simulink model "untitled"  (R2023a)
settings: Solver=VariableStepAuto  StartTime=0.0  StopTime=10.0  RelTol=1e-3
(part 2 of 2)

== system untitled/Subsystem/AdjustingStage/Normalizer/EightBitComparator/FourBitComparator ==
  In1 : Inport
  In2 : Inport  Port=2
  In3 : Inport  Port=3
  In5 : Inport  Port=4
  In4 : Inport  Port=5
  FourBitComparator : Subsystem
  Out1 : Outport
  Out2 : Outport  Port=2
  Out3 : Outport  Port=3

== system untitled/Subsystem/AdjustingStage/Normalizer/EightBitComparator/FourBitComparator1 ==
  In1 : Inport
  In2 : Inport  Port=2
  In3 : Inport  Port=3
  In5 : Inport  Port=4
  In4 : Inport  Port=5
  Out1 : Outport
  Out2 : Outport  Port=2
  Out3 : Outport  Port=3

== system untitled/Subsystem/AdjustingStage/Normalizer/EightBitComparator/Subsystem ==
  In1 : Inport
  Out1 : Outport
  wires:
  In1/1 -> Out1/1

== system untitled/Subsystem/AdjustingStage/Normalizer/EightBitComparator/Subsystem1 ==
  In1 : Inport
  Out1 : Outport
  wires:
  In1/1 -> Out1/1

== system untitled/Subsystem/AdjustingStage/Normalizer/EightBitComparator/Subsystem2 ==
  In1 : Inport
  Out1 : Outport
  wires:
  In1/1 -> Out1/1

== system untitled/Subsystem/AdjustingStage/Normalizer/EightBitComparator/Subsystem3 ==
  In1 : Inport
  Out1 : Outport
  wires:
  In1/1 -> Out1/1

== system untitled/Subsystem/ComparingStage/Comparator/EightBitComparator/FourBitComparator ==
  In1 : Inport
  In2 : Inport  Port=2
  In3 : Inport  Port=3
  In5 : Inport  Port=4
  In4 : Inport  Port=5
  Out1 : Outport
  Out2 : Outport  Port=2
  Out3 : Outport  Port=3

== system untitled/Subsystem/ComparingStage/Comparator/EightBitComparator/FourBitComparator1 ==
  In1 : Inport
  In2 : Inport  Port=2
  In3 : Inport  Port=3
  In5 : Inport  Port=4
  In4 : Inport  Port=5
  Out1 : Outport
  Out2 : Outport  Port=2
  Out3 : Outport  Port=3

== system untitled/Subsystem/ComparingStage/Comparator/EightBitComparator/Subsystem ==
  In1 : Inport
  Out1 : Outport
  wires:
  In1/1 -> Out1/1

== system untitled/Subsystem/ComparingStage/Comparator/EightBitComparator/Subsystem1 ==
  In1 : Inport
  Out1 : Outport
  wires:
  In1/1 -> Out1/1

== system untitled/Subsystem/ComparingStage/Comparator/EightBitComparator/Subsystem2 ==
  In1 : Inport
  Out1 : Outport
  wires:
  In1/1 -> Out1/1

== system untitled/Subsystem/ComparingStage/Comparator/EightBitComparator/Subsystem3 ==
  In1 : Inport
  Out1 : Outport
  wires:
  In1/1 -> Out1/1

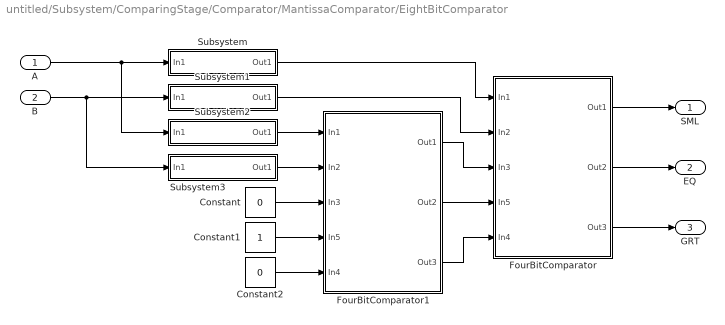
== system untitled/Subsystem/ComparingStage/Comparator/MantissaComparator/EightBitComparator ==
  A : Inport
  B : Inport  Port=2
  Constant : Constant  Value=0
  Constant1 : Constant
  Constant2 : Constant  Value=0
  FourBitComparator : Subsystem
      mask Display:
      | port_label('output', 1, 'SML_OUT');
      | port_label('output', 2, 'EQ_OUT');
      | port_label('output', 3, 'GRT_OUT');
      | port_label('input', 3, 'SML_IN');
      | port_label('input', 4, 'EQ_IN');
      | port_label('input', 5, 'GRT_IN');
  FourBitComparator1 : Subsystem
      mask Display:
      | port_label('output', 1, 'SML_OUT');
      | port_label('output', 2, 'EQ_OUT');
      | port_label('output', 3, 'GRT_OUT');
      | port_label('input', 3, 'SML_IN');
      | port_label('input', 4, 'EQ_IN');
      | port_label('input', 5, 'GRT_IN');
  Subsystem : Subsystem
      mask Display: disp('A(7 downto 4)');
  Subsystem1 : Subsystem
      mask Display: disp('B(7 downto 4)');
  Subsystem2 : Subsystem
      mask Display: disp('A(3 downto 0)');
  Subsystem3 : Subsystem
      mask Display: disp('B(3 downto 0)');
  SML : Outport
  EQ : Outport  Port=2
  GRT : Outport  Port=3
  wires:
  Subsystem3/1(Out1) -> FourBitComparator1/2(In2)
  Subsystem2/1(Out1) -> FourBitComparator1/1(In1)
  A/1 -> Subsystem2/1(In1), Subsystem/1(In1)
  B/1 -> Subsystem3/1(In1), Subsystem1/1(In1)
  Constant/1 -> FourBitComparator1/3(In3)
  Constant1/1 -> FourBitComparator1/4(In5)
  Constant2/1 -> FourBitComparator1/5(In4)
  Subsystem/1(Out1) -> FourBitComparator/1(In1)
  Subsystem1/1(Out1) -> FourBitComparator/2(In2)
  FourBitComparator1/1(Out1) -> FourBitComparator/3(In3)
  FourBitComparator1/2(Out2) -> FourBitComparator/4(In5)
  FourBitComparator1/3(Out3) -> FourBitComparator/5(In4)
  FourBitComparator/1(Out1) -> SML/1
  FourBitComparator/2(Out2) -> EQ/1
  FourBitComparator/3(Out3) -> GRT/1

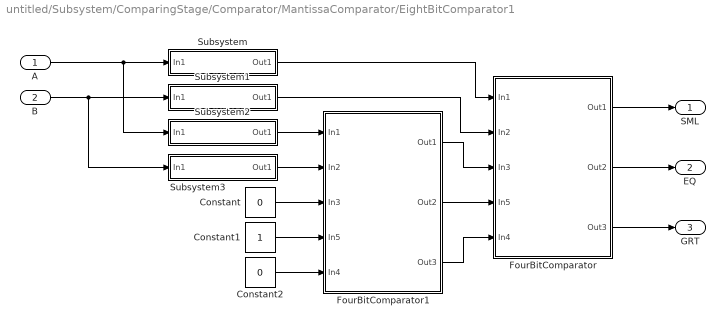
== system untitled/Subsystem/ComparingStage/Comparator/MantissaComparator/EightBitComparator1 ==
  A : Inport
  B : Inport  Port=2
  Constant : Constant  Value=0
  Constant1 : Constant
  Constant2 : Constant  Value=0
  FourBitComparator : Subsystem
      mask Display:
      | port_label('output', 1, 'SML_OUT');
      | port_label('output', 2, 'EQ_OUT');
      | port_label('output', 3, 'GRT_OUT');
      | port_label('input', 3, 'SML_IN');
      | port_label('input', 4, 'EQ_IN');
      | port_label('input', 5, 'GRT_IN');
  FourBitComparator1 : Subsystem
      mask Display:
      | port_label('output', 1, 'SML_OUT');
      | port_label('output', 2, 'EQ_OUT');
      | port_label('output', 3, 'GRT_OUT');
      | port_label('input', 3, 'SML_IN');
      | port_label('input', 4, 'EQ_IN');
      | port_label('input', 5, 'GRT_IN');
  Subsystem : Subsystem
      mask Display: disp('A(7 downto 4)');
  Subsystem1 : Subsystem
      mask Display: disp('B(7 downto 4)');
  Subsystem2 : Subsystem
      mask Display: disp('A(3 downto 0)');
  Subsystem3 : Subsystem
      mask Display: disp('B(3 downto 0)');
  SML : Outport
  EQ : Outport  Port=2
  GRT : Outport  Port=3
  wires:
  Subsystem3/1(Out1) -> FourBitComparator1/2(In2)
  Subsystem2/1(Out1) -> FourBitComparator1/1(In1)
  A/1 -> Subsystem2/1(In1), Subsystem/1(In1)
  B/1 -> Subsystem3/1(In1), Subsystem1/1(In1)
  Constant/1 -> FourBitComparator1/3(In3)
  Constant1/1 -> FourBitComparator1/4(In5)
  Constant2/1 -> FourBitComparator1/5(In4)
  Subsystem/1(Out1) -> FourBitComparator/1(In1)
  Subsystem1/1(Out1) -> FourBitComparator/2(In2)
  FourBitComparator1/1(Out1) -> FourBitComparator/3(In3)
  FourBitComparator1/2(Out2) -> FourBitComparator/4(In5)
  FourBitComparator1/3(Out3) -> FourBitComparator/5(In4)
  FourBitComparator/1(Out1) -> SML/1
  FourBitComparator/2(Out2) -> EQ/1
  FourBitComparator/3(Out3) -> GRT/1

== system untitled/Subsystem/ComparingStage/Comparator/MantissaComparator/EightBitComparator2 ==
  A : Inport
  B : Inport  Port=2
  Constant : Constant  Value=0
  Constant1 : Constant
  Constant2 : Constant  Value=0
  FourBitComparator : Subsystem
      mask Display:
      | port_label('output', 1, 'SML_OUT');
      | port_label('output', 2, 'EQ_OUT');
      | port_label('output', 3, 'GRT_OUT');
      | port_label('input', 3, 'SML_IN');
      | port_label('input', 4, 'EQ_IN');
      | port_label('input', 5, 'GRT_IN');
  FourBitComparator1 : Subsystem
      mask Display:
      | port_label('output', 1, 'SML_OUT');
      | port_label('output', 2, 'EQ_OUT');
      | port_label('output', 3, 'GRT_OUT');
      | port_label('input', 3, 'SML_IN');
      | port_label('input', 4, 'EQ_IN');
      | port_label('input', 5, 'GRT_IN');
  Subsystem : Subsystem
      mask Display: disp('A(7 downto 4)');
  Subsystem1 : Subsystem
      mask Display: disp('B(7 downto 4)');
  Subsystem2 : Subsystem
      mask Display: disp('A(3 downto 0)');
  Subsystem3 : Subsystem
      mask Display: disp('B(3 downto 0)');
  SML : Outport
  EQ : Outport  Port=2
  GRT : Outport  Port=3
  wires:
  Subsystem3/1(Out1) -> FourBitComparator1/2(In2)
  Subsystem2/1(Out1) -> FourBitComparator1/1(In1)
  A/1 -> Subsystem2/1(In1), Subsystem/1(In1)
  B/1 -> Subsystem3/1(In1), Subsystem1/1(In1)
  Constant/1 -> FourBitComparator1/3(In3)
  Constant1/1 -> FourBitComparator1/4(In5)
  Constant2/1 -> FourBitComparator1/5(In4)
  Subsystem/1(Out1) -> FourBitComparator/1(In1)
  Subsystem1/1(Out1) -> FourBitComparator/2(In2)
  FourBitComparator1/1(Out1) -> FourBitComparator/3(In3)
  FourBitComparator1/2(Out2) -> FourBitComparator/4(In5)
  FourBitComparator1/3(Out3) -> FourBitComparator/5(In4)
  FourBitComparator/1(Out1) -> SML/1
  FourBitComparator/2(Out2) -> EQ/1
  FourBitComparator/3(Out3) -> GRT/1

== system untitled/Subsystem/ComparingStage/Comparator/MantissaComparator/FourBitComparator ==
  In1 : Inport
  In2 : Inport  Port=2
  In3 : Inport  Port=3
  In5 : Inport  Port=4
  In4 : Inport  Port=5
  Out1 : Outport
  Out2 : Outport  Port=2
  Out3 : Outport  Port=3

== system untitled/Subsystem/ComparingStage/Comparator/MantissaComparator/Subsystem ==
  In1 : Inport
  In2 : Inport  Port=2
  In3 : Inport  Port=3
  Out1 : Outport
  wires:
  In1/1 -> Out1/1

== system untitled/Subsystem/ComparingStage/Comparator/MantissaComparator/Subsystem1 ==
  In1 : Inport
  In2 : Inport  Port=2
  In3 : Inport  Port=3
  Out1 : Outport
  wires:
  In1/1 -> Out1/1

== system untitled/Subsystem/ComparingStage/Comparator/MantissaComparator/Subsystem2 ==
  In1 : Inport
  Out1 : Outport
  wires:
  In1/1 -> Out1/1

== system untitled/Subsystem/ComparingStage/Comparator/MantissaComparator/Subsystem3 ==
  In1 : Inport
  Out1 : Outport
  wires:
  In1/1 -> Out1/1

== system untitled/Subsystem/ComparingStage/Comparator/MantissaComparator/Subsystem4 ==
  In1 : Inport
  Out1 : Outport
  wires:
  In1/1 -> Out1/1

== system untitled/Subsystem/ComparingStage/Comparator/MantissaComparator/Subsystem5 ==
  In1 : Inport
  Out1 : Outport
  wires:
  In1/1 -> Out1/1

== system untitled/Subsystem/ComparingStage/Comparator/MantissaComparator/Subsystem6 ==
  In1 : Inport
  Out1 : Outport
  wires:
  In1/1 -> Out1/1

== system untitled/Subsystem/ComparingStage/Comparator/MantissaComparator/Subsystem7 ==
  In1 : Inport
  Out1 : Outport
  wires:
  In1/1 -> Out1/1

== system untitled/Subsystem/AdjustingStage/Normalizer/EightBitComparator/FourBitComparator/FourBitComparator ==
  A : Inport
  B : Inport  Port=2
  SML_IN : Inport  Port=3
  EQ_IN : Inport  Port=4
  GRT_IN : Inport  Port=5
  SML_OUT : Outport
  EQ_OUT : Outport  Port=2
  GRT_OUT : Outport  Port=3
  wires:
  A/1 -> SML_OUT/1

== system untitled/Subsystem/ComparingStage/Comparator/MantissaComparator/EightBitComparator/FourBitComparator ==
  In1 : Inport
  In2 : Inport  Port=2
  In3 : Inport  Port=3
  In5 : Inport  Port=4
  In4 : Inport  Port=5
  Out1 : Outport
  Out2 : Outport  Port=2
  Out3 : Outport  Port=3

== system untitled/Subsystem/ComparingStage/Comparator/MantissaComparator/EightBitComparator/FourBitComparator1 ==
  In1 : Inport
  In2 : Inport  Port=2
  In3 : Inport  Port=3
  In5 : Inport  Port=4
  In4 : Inport  Port=5
  Out1 : Outport
  Out2 : Outport  Port=2
  Out3 : Outport  Port=3

== system untitled/Subsystem/ComparingStage/Comparator/MantissaComparator/EightBitComparator/Subsystem ==
  In1 : Inport
  Out1 : Outport
  wires:
  In1/1 -> Out1/1

== system untitled/Subsystem/ComparingStage/Comparator/MantissaComparator/EightBitComparator/Subsystem1 ==
  In1 : Inport
  Out1 : Outport
  wires:
  In1/1 -> Out1/1

== system untitled/Subsystem/ComparingStage/Comparator/MantissaComparator/EightBitComparator/Subsystem2 ==
  In1 : Inport
  Out1 : Outport
  wires:
  In1/1 -> Out1/1

== system untitled/Subsystem/ComparingStage/Comparator/MantissaComparator/EightBitComparator/Subsystem3 ==
  In1 : Inport
  Out1 : Outport
  wires:
  In1/1 -> Out1/1

== system untitled/Subsystem/ComparingStage/Comparator/MantissaComparator/EightBitComparator1/FourBitComparator ==
  In1 : Inport
  In2 : Inport  Port=2
  In3 : Inport  Port=3
  In5 : Inport  Port=4
  In4 : Inport  Port=5
  Out1 : Outport
  Out2 : Outport  Port=2
  Out3 : Outport  Port=3

== system untitled/Subsystem/ComparingStage/Comparator/MantissaComparator/EightBitComparator1/FourBitComparator1 ==
  In1 : Inport
  In2 : Inport  Port=2
  In3 : Inport  Port=3
  In5 : Inport  Port=4
  In4 : Inport  Port=5
  Out1 : Outport
  Out2 : Outport  Port=2
  Out3 : Outport  Port=3

== system untitled/Subsystem/ComparingStage/Comparator/MantissaComparator/EightBitComparator1/Subsystem ==
  In1 : Inport
  Out1 : Outport
  wires:
  In1/1 -> Out1/1

== system untitled/Subsystem/ComparingStage/Comparator/MantissaComparator/EightBitComparator1/Subsystem1 ==
  In1 : Inport
  Out1 : Outport
  wires:
  In1/1 -> Out1/1

== system untitled/Subsystem/ComparingStage/Comparator/MantissaComparator/EightBitComparator1/Subsystem2 ==
  In1 : Inport
  Out1 : Outport
  wires:
  In1/1 -> Out1/1

== system untitled/Subsystem/ComparingStage/Comparator/MantissaComparator/EightBitComparator1/Subsystem3 ==
  In1 : Inport
  Out1 : Outport
  wires:
  In1/1 -> Out1/1

== system untitled/Subsystem/ComparingStage/Comparator/MantissaComparator/EightBitComparator2/FourBitComparator ==
  In1 : Inport
  In2 : Inport  Port=2
  In3 : Inport  Port=3
  In5 : Inport  Port=4
  In4 : Inport  Port=5
  Out1 : Outport
  Out2 : Outport  Port=2
  Out3 : Outport  Port=3

== system untitled/Subsystem/ComparingStage/Comparator/MantissaComparator/EightBitComparator2/FourBitComparator1 ==
  In1 : Inport
  In2 : Inport  Port=2
  In3 : Inport  Port=3
  In5 : Inport  Port=4
  In4 : Inport  Port=5
  Out1 : Outport
  Out2 : Outport  Port=2
  Out3 : Outport  Port=3

== system untitled/Subsystem/ComparingStage/Comparator/MantissaComparator/EightBitComparator2/Subsystem ==
  In1 : Inport
  Out1 : Outport
  wires:
  In1/1 -> Out1/1

== system untitled/Subsystem/ComparingStage/Comparator/MantissaComparator/EightBitComparator2/Subsystem1 ==
  In1 : Inport
  Out1 : Outport
  wires:
  In1/1 -> Out1/1

== system untitled/Subsystem/ComparingStage/Comparator/MantissaComparator/EightBitComparator2/Subsystem2 ==
  In1 : Inport
  Out1 : Outport
  wires:
  In1/1 -> Out1/1

== system untitled/Subsystem/ComparingStage/Comparator/MantissaComparator/EightBitComparator2/Subsystem3 ==
  In1 : Inport
  Out1 : Outport
  wires:
  In1/1 -> Out1/1
